simulink model "lab_modulation_pm"  (R2024b)
settings: Solver=FixedStepDiscrete  StartTime=0.0  StopTime=1  FixedStep=0.0001  RelTol=1e-3
model workspace (MAT data in the model file):
  Sig = Simulink.Signal
  Sig.Dimensions = -1
  Sig.DimensionsMode = 'auto'
  Sig.Complexity = 'auto'
  Sig.SampleTime = -1
  Sig.SamplingMode = 'auto'
  Sig.DataType = 'auto'
  phaseDeviation = 0.785398163397
  variance = 0
libraries: dspfdesign x1, commanapbnd3 x1
settings Model: Creator=andrey  LastModifiedBy=andrey

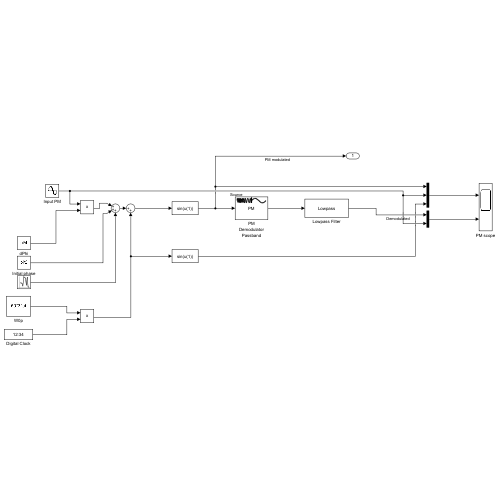
[thumbnail: Simulink's stored preview of the top-level diagram]
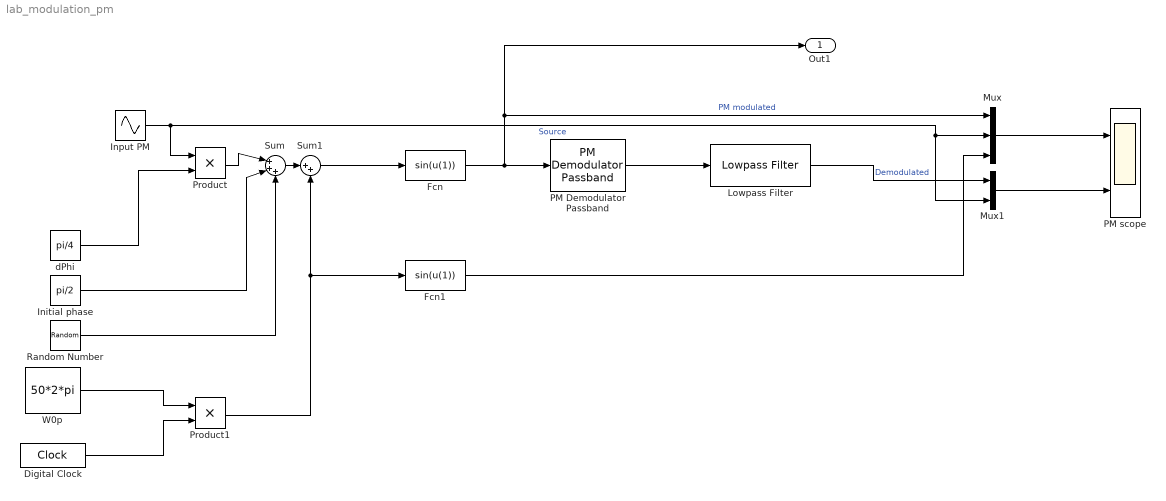
== system lab_modulation_pm ==
  Digital Clock : DigitalClock  SampleTime=0.0001
  Fcn : Fcn  Expr=sin(u(1))
  Fcn1 : Fcn  Expr=sin(u(1))
  Initial phase : Constant  Value=pi/2
  Input PM : Sin  Frequency=2*2*pi  SampleTime=0.0001
  Lowpass Filter : dspfdesign/Lowpass Filter  FilterType=FIR  DesignForMinimumOrder=on  FilterOrder=50  PassbandFrequency=0.1  StopbandFrequency=100  PassbandRipple=0.1  StopbandAttenuation=80  SampleRate=44100  SimulateUsing=Interpreted execution  roundingMode=Floor  coeffsDataTypeStr=fixdt(1,16)
  Mux : Mux  Inputs=3
  Mux1 : Mux  Inputs=2
  PM Demodulator Passband : commanapbnd3/PM Demodulator Passband  Fc=50  Ph=0  Kc=phaseDeviation  Ho=100
  PM scope : Scope  NumInputPorts=2
  Product : Product
  Product1 : Product
  Random Number : RandomNumber  Mean=0.5  Variance=variance  SampleTime=0.0001
  Sum : Sum  Inputs=|+++
  Sum1 : Sum  Inputs=|++
  W0p : Constant  Value=50*2*pi
  dPhi : Constant  Value=pi/4
  Out1 : Outport
  wires:
  Input PM/1 -> Mux1/2, Mux/2, Product/1  "Source"
  Mux/1 -> PM scope/1
  dPhi/1 -> Product/2
  Product/1 -> Sum/1
  Initial phase/1 -> Sum/2
  Mux1/1 -> PM scope/2
  Lowpass Filter/1 -> Mux1/1  "Demodulated"
  W0p/1 -> Product1/1
  Digital Clock/1 -> Product1/2
  Sum/1 -> Sum1/1
  Product1/1 -> Fcn1/1, Sum1/2
  Sum1/1 -> Fcn/1
  Fcn/1 -> Out1/1, Mux/1, PM Demodulator Passband/1  "PM modulated"
  PM Demodulator Passband/1 -> Lowpass Filter/1
  Fcn1/1 -> Mux/3
  Random Number/1 -> Sum/3
